simulink model "P4_simulink2022a"  (R2022a)
settings: Solver=VariableStepAuto  StartTime=0.0  StopTime=10.0  RelTol=1e-10
values from neighbouring files (symbols this model uses):
  Altura = 100    [P2.m]    (also in P3.m = 10; P4.m = 10; TestGraph.m = 10; ZenoPlot.m = 10)
  K = -0.8    [P1.m]    (also in P2.m = -1; P4.m; TestGraph.m; ZenoPlot.m)
  V = 0    [P1.m]    (also in P2.m = 15; P3.m = 15; P4.m = 15; QuiverTest.m = zeros(length(U),length(U)) -g)
libraries: simulink x2
settings Model: Creator=TERESA NOGUEIRA  LastModifiedBy=TERESA NOGUEIRA
settings SolverCC: ZeroCrossAlgorithm=Adaptive
settings ModelReferenceCC: EnableRefExpFcnMdlSchedulingChecks=off
settings RTWCC: Description=Generic Real-Time Target

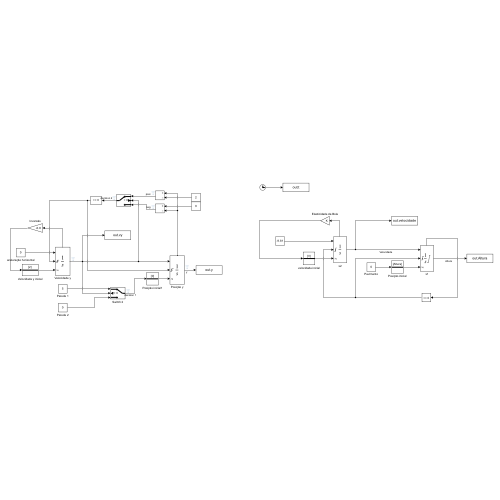
[thumbnail: Simulink's stored preview of the top-level diagram]
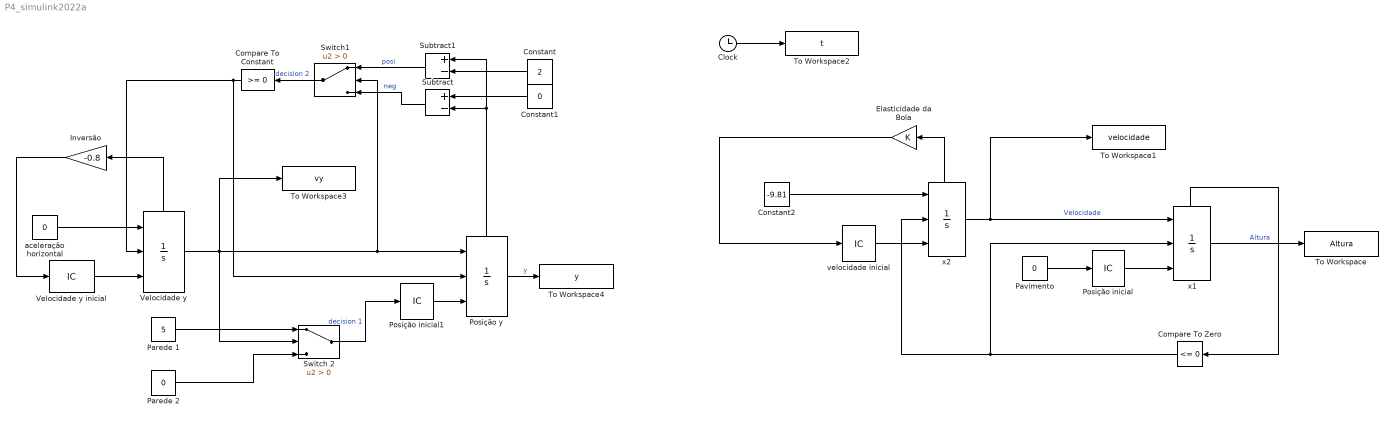
== system P4_simulink2022a ==
  Clock : Clock
      settings: Decimation=200
  Compare To Constant : simulink/Logic and Bit Operations/Compare To Constant  relop=>=  const=0  OutDataTypeStr=boolean
  Compare To Zero : simulink/Logic and Bit Operations/Compare To Zero  relop=<=  OutDataTypeStr=boolean
  Constant : Constant  Value=2
  Constant1 : Constant  Value=0
  Constant2 : Constant  Value=-9.81
  Elasticidade da Bola : Gain  Gain=K
  Inversão : Gain  Gain=-0.8
  Parede 1 : Constant  Value=5
  Parede 2 : Constant  Value=0
  Pavimento : Constant  Value=0
  Posição inicial : InitialCondition  Value=Altura
  Posição inicial1 : InitialCondition  Value=0
  Posição y : Integrator  ExternalReset=rising  InitialConditionSource=external  ShowStatePort=on
  Subtract : Sum  Inputs=+-
  Subtract1 : Sum  Inputs=+-
  Switch 2 : Switch  Criteria=u2 > Threshold  SaturateOnIntegerOverflow=off  InputSameDT=off
  Switch1 : Switch  Criteria=u2 > Threshold  SaturateOnIntegerOverflow=off  InputSameDT=off
  To Workspace : ToWorkspace  VariableName=Altura  SampleTime=-1
      settings: Save2DSignal=2-D array (concatenate along first dimension)
  To Workspace1 : ToWorkspace  VariableName=velocidade  SampleTime=-1
      settings: Save2DSignal=2-D array (concatenate along first dimension)
  To Workspace2 : ToWorkspace  VariableName=t  SampleTime=-1
      settings: Save2DSignal=2-D array (concatenate along first dimension)
  To Workspace3 : ToWorkspace  VariableName=vy  SampleTime=-1
  To Workspace4 : ToWorkspace  VariableName=y  SampleTime=-1
  Velocidade y : Integrator  ExternalReset=rising  InitialConditionSource=external  ShowStatePort=on
  Velocidade y inicial : InitialCondition  Value=2
  aceleração horizontal : Constant  Value=0
  velocidade inicial : InitialCondition  Value=V
  x1 : Integrator  ExternalReset=rising  InitialConditionSource=external  LimitOutput=on  LowerSaturationLimit=0  ShowStatePort=on
  x2 : Integrator  ExternalReset=rising  InitialConditionSource=external  ShowStatePort=on
  wires:
  Velocidade y inicial/1 -> Velocidade y/3
  Inversão/1 -> Velocidade y inicial/1
  Compare To Constant/1 -> Velocidade y/2, Posição y/2
  aceleração horizontal/1 -> Velocidade y/1
  Posição inicial1/1 -> Posição y/3
  Velocidade y/1 -> To Workspace3/1, Switch1/2, Posição y/1, Switch 2/2
  Posição y/1 -> To Workspace4/1  "y"
  Velocidade y/State -> Inversão/1
  Posição y/State -> Subtract1/1, Subtract/2
  Switch 2/1 -> Posição inicial1/1  "decision 1"
  Parede 2/1 -> Switch 2/3
  Parede 1/1 -> Switch 2/1
  Constant/1 -> Subtract1/2
  Constant1/1 -> Subtract/1
  Switch1/1 -> Compare To Constant/1  "decision 2"
  Subtract/1 -> Switch1/3  "neg"
  Subtract1/1 -> Switch1/1  "posi"
  x2/1 -> To Workspace1/1, x1/1  "Velocidade"
  x1/1 -> To Workspace/1  "Altura"
  velocidade inicial/1 -> x2/3
  Compare To Zero/1 -> x2/2, x1/2
  Constant2/1 -> x2/1
  Clock/1 -> To Workspace2/1
  Posição inicial/1 -> x1/3
  x2/State -> Elasticidade da Bola/1
  x1/State -> Compare To Zero/1
  Elasticidade da Bola/1 -> velocidade inicial/1
  Pavimento/1 -> Posição inicial/1
